simulink model "Testabc_dq"  (R2023b)
settings: Solver=VariableStepAuto  StartTime=0.0  StopTime=10.0  RelTol=1e-3
libraries: spsabctodq0Lib x1
settings Model: Creator=snow_  LastModifiedBy=snow_

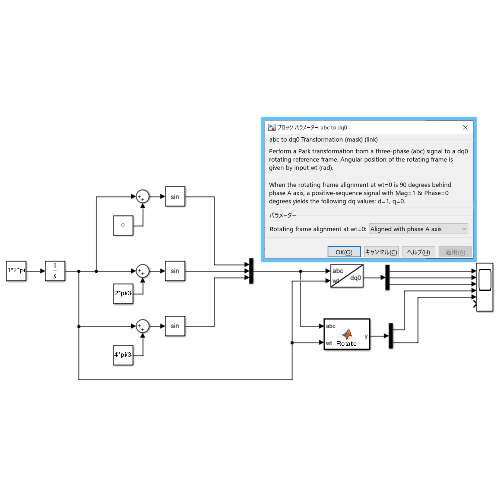
[thumbnail: Simulink's stored preview of the top-level diagram]
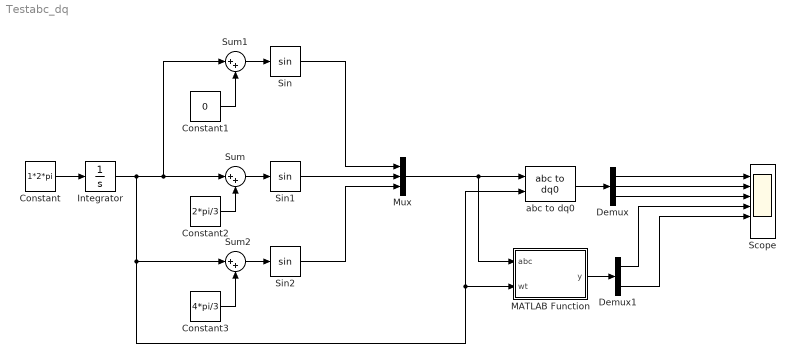
== system Testabc_dq ==
  Constant : Constant  Value=1*2*pi
  Constant1 : Constant  Value=0
  Constant2 : Constant  Value=2*pi/3
  Constant3 : Constant  Value=4*pi/3
  Demux : Demux  Outputs=3
  Demux1 : Demux  Outputs=2
  Integrator : Integrator
  MATLAB Function : MATLAB Function  TreatAsAtomicUnit=on
  Mux : Mux  Inputs=3
  Scope : Scope  NumInputPorts=6
  Sin : Trigonometry
  Sin1 : Trigonometry
  Sin2 : Trigonometry
  Sum : Sum  Inputs=|++
  Sum1 : Sum  Inputs=|++
  Sum2 : Sum  Inputs=|++
  abc to dq0 : spsabctodq0Lib/abc to dq0  Alignment=Aligned with phase A axis
  wires:
  Constant/1 -> Integrator/1
  Sum1/1 -> Sin/1
  Sum/1 -> Sin1/1
  Sum2/1 -> Sin2/1
  Constant1/1 -> Sum1/2
  Constant3/1 -> Sum2/2
  Constant2/1 -> Sum/2
  Sin/1 -> Mux/1
  Sin1/1 -> Mux/2
  Sin2/1 -> Mux/3
  Integrator/1 -> Sum2/1, MATLAB Function/2(wt), abc to dq0/2, Sum/1, Sum1/1
  Mux/1 -> MATLAB Function/1(abc), abc to dq0/1
  abc to dq0/1 -> Demux/1
  Demux/1 -> Scope/1
  Demux/2 -> Scope/2
  Demux/3 -> Scope/3
  Demux1/1 -> Scope/4
  Demux1/2 -> Scope/5
  MATLAB Function/1(y) -> Demux1/1

== matlab function Testabc_dq/MATLAB Function ==
  data: abc input; y output; wt input
function y = Rotate(abc,wt)

C = [cos(wt) cos(wt-2/3*pi) cos(wt-4/3*pi);
    -1*sin(wt) -1*sin(wt-2/3*pi) -1*sin(wt-4/3*pi)];

y = sqrt(2/3)*C*[abc(1);abc(2);abc(3)];
